simulink model "vnsimulink"  (R2020a)
settings: Solver=ode4  StartTime=0.0  StopTime=20  FixedStep=8e-6  RelTol=1e-3
undefined symbols (not defined in the file or in its folder): D1, Delta, sigbuilder_block
libraries: powerlib x98, powerlib_meascontrol x21, simulink x16
(part 3 of 3)

== system vnsimulink/PV15kW2/Subsystem/Subsystem/Power Loop2 ==
  vp : Inport
  vn : Inport  Port=2
  av : Inport  Port=3
  ip : Inport  Port=4
  outn : Inport  Port=5
  Trigger : TriggerPort  VariantControl=(inherit)
  Pcut-sim1 : MATLAB Function  TreatAsAtomicUnit=on
  Pmax-sim2 : MATLAB Function  TreatAsAtomicUnit=on
  Scope : Scope
  m : Outport
  m2 : Outport  Port=2
  m3 : Outport  Port=3
  m4 : Outport  Port=4
  wires:
  vp/1 -> Pmax-sim2/1(vp)
  vn/1 -> Pmax-sim2/2(vn)
  av/1 -> Pmax-sim2/3(av)
  ip/1 -> Pmax-sim2/4(ip)
  outn/1 -> Pmax-sim2/5(outn)
  Pmax-sim2/1(gn) -> m/1
  Pmax-sim2/2(phi) -> m2/1
  Pmax-sim2/3(kii) -> m3/1
  Pmax-sim2/4(ppv) -> m4/1
  Pmax-sim2/5(x) -> Scope/1

== system vnsimulink/PV15kW2/Subsystem/Subsystem2/integral  ==
  di : Inport
  kii : Inport  Port=2
  gmax : Inport  Port=3
  Trigger : TriggerPort  VariantControl=(inherit)
  Embedded MATLAB Function : MATLAB Function  TreatAsAtomicUnit=on
  w : Outport
  wires:
  Embedded MATLAB Function/1(w) -> w/1
  di/1 -> Embedded MATLAB Function/1(di)
  kii/1 -> Embedded MATLAB Function/2(kii)
  gmax/1 -> Embedded MATLAB Function/3(gmax)

== system vnsimulink/PV15kW2/Subsystem/Subsystem8/GIVF ==
  Vgq : Inport
  Trigger : TriggerPort  VariantControl=(inherit)
  Embedded MATLAB Function : MATLAB Function  TreatAsAtomicUnit=on
  Out1 : Outport
  y2 : Outport  Port=2
  wires:
  Embedded MATLAB Function/1(y1) -> Out1/1
  Vgq/1 -> Embedded MATLAB Function/1(u)
  Embedded MATLAB Function/2(y2) -> y2/1

== system vnsimulink/PV15kW2/Subsystem/Subsystem9/GIVF ==
  Vgq : Inport
  Trigger : TriggerPort  VariantControl=(inherit)
  Embedded MATLAB Function : MATLAB Function  TreatAsAtomicUnit=on
  Out1 : Outport
  y2 : Outport  Port=2
  wires:
  Embedded MATLAB Function/1(y1) -> Out1/1
  Vgq/1 -> Embedded MATLAB Function/1(u)
  Embedded MATLAB Function/2(y2) -> y2/1

== matlab function vnsimulink/PV15kW2/Subsystem/Subsystem/Power Loop2/Pcut-sim1 ==
  data: vp input; vn input; av input; gn output; phi output; ip input; outn input; kii output; ppv output
function [gn,phi,kii,ppv] = Algorithm(vp,vn,av,ip,outn)

ilim=41;
d=0.6;ppv=15060;
persistent flag D Dold ppvold ppv1
persistent ca ir i ki ctc
persistent m sum1 sum2 ipo an
persistent vns vps up un un0 un1 uns kn kn0 kns kn1 
persistent outns outn0 outn1 on m1 m2
persistent a1 b1 c1 a2 b2 c2 a3 b3 c3 kna knb knc A B C 
dataType = 'double';
%initial
if isempty(D)
flag=1;D=1;Dold=1;
ca=0;ir=0;i=0;ctc=0;
ipo=0;m=0;sum1=40;sum2=14;an=0;
vns=0;vps=0;ppvold=15000;ppv1=15000;
un=0;un0=0;un1=0;uns=0;kn=0;kn0=0;kns=0;kn1=0;
outns=0;outn0=0;outn1=0;on=0;m1=0;m2=0;ki=1;
a1=0;b1=0;c1=0;a2=0;b2=0;c2=0;a3=0;b3=0;c3=0;kna=0;knb=0;knc=0;A=0;B=0;C=0;
end
ctc=ctc+1;

if sum1>0
    sum1=sum1-1;
    vns=vns+vn;vps=vps+vp;
end
if sum1==0
sum1=40;
% vns=vns+vn;vps=vps+vp;
un=vns/40;up=vps/40;
vns=0;vps=0;

% no p limit
if flag==1
    un1=un;flag=0;kn=0;m=185;
else
    
if sum2==0
    sum2=14;
    un0=(uns+un)/11;
    outn0=(outns+outn)/11;
    kn0=(kns+kn)/11;

%PV power change?
  if (abs(ip-ipo)>0.1)
  ir=1;
  else
  ir=0;
  end
%select case
ca=0;ki=1;
if (ir==0)
  if (on==1)
      ca=1;end
  if (on==0)   
      ca=2;end 
  if (outn<kn)&&(un0<1.63)
      ca=3;end
%case1 
  if (ca==1)
   %power curtail
   vnx=2;
   zn=0.368;thv=37;vn0=7.11;
   if ctc>30600
   zn=0.373;thv=42.5;vn0=7.61;end
   if ctc>81000
   zn=0.4068;thv=43.4;vn0=8.27;end   
   %mp=th2-th1+atan(0.65)-pi;
   ipm=sqrt((ilim*zn+vnx)^2-(vn0*sin(thv/180*pi))^2)-vn0*cos(thv/180*pi);
   ppvn=1.5*ipm/zn*vp-1.5*vn*vn*kn;
   th1=pi-asin(vn0*sin(thv/180*pi)/(ilim*zn+vnx));
   xp=-ilim*zn/(sqrt(1+(vn0*sin(thv/180*pi)/(ilim*zn+vnx))^2));
   yp=-xp*vn0*sin(thv/180*pi)/(ilim*zn+vnx);
   th2=2*pi-atan(yp/(-xp-ipm));
   mp=th2-2/3*pi; 
   %exit curtail
    if abs(ppvold-ppvn)<75
    ppvn=ppvold;
    else
    m=mp*180/pi;
    ca=0;
    end
    ppv1=ppvn;
    ppvold=ppv1;
  end
  if (ca==1)    
   if Dold==1
    if un0>un1
      D=-1;
    else
      D=1;
    end
   else
    if un0>un1
      D=1;
    else
      D=-1;
    end 
   end
  end
%case2 
  if ca==2
    if (un0>1.003*un1)
    ca=2;ki=0;
    else
    ca=0;    
    end
  end
%case3
 if (ca==3)
  if Dold==1
   if un0*outn0>un1*outn1
      D=-1;
   else
      D=1;
   end
  else
   if un0*outn0>un1*outn1
      D=1;
   else
      D=-1;
   end 
  end
 end
%update D
 if (ca==1)||(ca==2)||(ca==3)
  Dold=D;
   if D==-1   
      m=m-d;
   else
      m=m+d;
   end
  end  
end
%%exit case
 un1=un0;outn1=outn0;kn1=kn0;ipo=ip;m2=m1;m1=m;
%%sum!=0
else
    if (sum2<=10)
        i=1;
    else
        i=2;
        if (sum2>10)
        i=0;
        end
    end
    if i==1
    uns=uns+un;outns=outns+outn;kns=kns+kn;sum2=sum2-1;i=3;
     if outn>kn
        on=1;end
    end
    if i==0
    uns=0;outns=0;kns=0;sum2=sum2-1;i=3;on=0;
     if outn>kn
        on=1;end
    end
    if i==2
    sum2=sum2-1;i=3;
     if outn>kn
        on=1;
     end
    end
end

%%current limit
     an=m/180*pi;
    a1=vn^2;
    b1=2*ip*un*cos(an);
    c1=ip^2-ilim^2;
kna=(-b1+sqrt(b1^2-4*a1*c1))/(2*a1);
    a3=vn^2;
    b3=2*ip*un*cos(an-pi*2/3);
    c3=ip^2-ilim^2;
knc=(-b3+sqrt(b3^2-4*a3*c3))/(2*a3);
    a2=vn^2;
    b2=2*ip*un*cos(an+pi*2/3);
    c2=ip^2-ilim^2;
knb=(-b2+sqrt(b2^2-4*a2*c2))/(2*a2);
kn=min(min(kna,knb),knc);
%power fluctuation
A=un^2*up^2;
B=2*un*up*ip*cos(av-an);
C=un^2*ip^2-(8000/1.5)^2;
knm=(-B+sqrt(B^2-4*A*C))/(2*A);
kn=min(kn,knm);
end
end
phi=m;gn=kn;kii=ki;ppv=ppv1;

== matlab function vnsimulink/PV15kW2/Subsystem/Subsystem2/integral /Embedded MATLAB Function ==
  data: di input; w output; kii input; gmax input
function w  = Algorithm(di,kii,gmax)

%控制器参数
T=20e-5;%控制周期
% ki1=3;
% ki2=3;
ki1=2.5;
ki2=12;
persistent sum ct;
dataType = 'double';

%首次赋值
if isempty(sum)
    sum=0;ct=0;
end

 if di>=0.2
 sum=kii*ki1*T*di+sum;
 else
 sum=kii*ki2*T*di+sum; 
 end
 
 if sum>1.1*gmax
     ct=ct+1;
     if ct==600
     ct=0;
     sum=1.07*gmax;
     end
 end   
   w=sum;

== matlab function vnsimulink/PV15kW2/Subsystem/Subsystem8/GIVF/Embedded MATLAB Function ==
  data: u input; y1 output; y2 output
function [y1,y2] = Algorithm(u)

%控制器参数
T=2e-4;k=314.1593;
persistent u0 u1 u2 u3 u4 u5;
dataType = 'double';

%首次赋值
if isempty(u0)
u0=0;u1=0;u2=0;u3=0;u4=0;u5=0;
end

u0=u;
u1=u0-u2-u3-u4;
u2=k*T*u1+u2;
u3=k*T*u2+u3;
u4=k*T*(0.5*u2-u5)+u4;
u5=k*T*u4+u5;
y1=0.5*u4;
y2=0.5*u5;
end

== matlab function vnsimulink/PV15kW2/Subsystem/Subsystem9/GIVF/Embedded MATLAB Function ==
  data: u input; y1 output; y2 output
function [y1,y2] = Algorithm(u)

%控制器参数
T=2e-4;k=314.1593;
persistent u0 u1 u2 u3 u4 u5;
dataType = 'double';

%首次赋值
if isempty(u0)
u0=0;u1=0;u2=0;u3=0;u4=0;u5=0;
end

u0=u;
u1=u0-u2-u3-u4;
u2=k*T*u1+u2;
u3=k*T*u2+u3;
u4=k*T*(0.5*u2-u5)+u4;
u5=k*T*u4+u5;
y1=0.5*u4;
y2=0.5*u5;
end

== matlab function vnsimulink/PV15kW2/Subsystem4/Power Loop1/Embedded MATLAB Function ==
  data: Vpv input; Ppv input; v output; l output; Pref input
function [v,l]= Algorithm(Vpv,Ppv,Pref)

%MPPT控制参数
v0 = 400;
vmax  = 600;
vmin = 200;
Deltav =0.1;


persistent Vpv_old Ppv_old v_old;
persistent flag nsum;


dataType = 'double';

%首次赋值
if isempty(Vpv_old)
    Vpv_old=0;
    Ppv_old=0;
    v_old=v0;
    flag=0;
    nsum=0;
end
% if nsum<(1.0/(20e-5))
%      flag=0;
% else
%      flag=1;
% end
% nsum=nsum+1;
% 
% if Vpv>800
%     flag=1;
% end
flag=1;
l=0;
if flag==1
%MPPT控制
dVpv=Vpv-Vpv_old;
dPpv=Ppv-Ppv_old;
if Ppv-Pref >= 0
    if dPpv >= 0
        if dVpv >= 0
            v = v_old + Deltav;%右侧
            l=11;
        else 
            v = v_old + Deltav;
            l=12;
        end
    else
        if dVpv >= 0
            v = v_old + Deltav;
            l=13;
        else
            v = v_old + Deltav;%右侧
            l=14;
        end
    end
else
    if dPpv >= 0
        if dVpv >=0
            v = v_old + Deltav;
             l=21;
        else
            v = v_old - Deltav;
             l=22;
        end
    else
        if dVpv >= 0
            v = v_old - Deltav;
             l=23;
        else
            v = v_old + Deltav;
             l=24;
        end
    end
end
% if Ppv-Pref >= 0
%      v = v_old - Deltav;
% else
%      v = v_old + Deltav;
% end
v_old=v;
Vpv_old=Vpv;
Ppv_old=Ppv;
else
 v=v0;   
end

== matlab function vnsimulink/PV15kW1/Subsystem/PLL/Embedded MATLAB Function ==
  data: Vgq input; w output
function w  = Algorithm(Vgq)

%控制器参数
T=20e-5;%控制周期

Kpllp=0.45;
Kplli=8;

persistent PLLsum;
persistent nsum2;

dataType = 'double';

%首次赋值
if isempty(PLLsum)
    PLLsum=0;
    nsum2=0;
end


w=Kpllp*Vgq+Kplli*(T*Vgq+PLLsum);
PLLsum=T*Vgq+PLLsum;
end

== matlab function vnsimulink/PV15kW2/Subsystem/PLL/Embedded MATLAB Function ==
  data: Vgq input; w output
function w  = Algorithm(Vgq)

%控制器参数
T=20e-5;%控制周期

Kpllp=0.45;
Kplli=8;

persistent PLLsum;
persistent nsum2;

dataType = 'double';

%首次赋值
if isempty(PLLsum)
    PLLsum=0;
    nsum2=0;
end


w=Kpllp*Vgq+Kplli*(T*Vgq+PLLsum);
PLLsum=T*Vgq+PLLsum;
end

== matlab function vnsimulink/PV15kW1/Subsystem/Subsystem/Power Loop2/Pcut-sim2 ==
  data: vp input; vn input; av input; gn output; phi output; ip input; outn input; kii output; ppv output
function [gn,phi,kii,ppv] = Algorithm(vp,vn,av,ip,outn)

ilim=41;
d=0.6;ppv=15060;
persistent flag D Dold ppvold ppv1
persistent ca ir i ki ctc
persistent m sum1 sum2 ipo an
persistent vns vps up un un0 un1 uns kn kn0 kns kn1 
persistent outns outn0 outn1 on m1 m2
persistent a1 b1 c1 a2 b2 c2 a3 b3 c3 kna knb knc A B C 
dataType = 'double';
%initial
if isempty(D)
flag=1;D=1;Dold=1;
ca=0;ir=0;i=0;ctc=0;
ipo=0;m=0;sum1=40;sum2=14;an=0;
vns=0;vps=0;ppvold=15000;ppv1=15000;
un=0;un0=0;un1=0;uns=0;kn=0;kn0=0;kns=0;kn1=0;
outns=0;outn0=0;outn1=0;on=0;m1=0;m2=0;ki=1;
a1=0;b1=0;c1=0;a2=0;b2=0;c2=0;a3=0;b3=0;c3=0;kna=0;knb=0;knc=0;A=0;B=0;C=0;
end
ctc=ctc+1;

if sum1>0
    sum1=sum1-1;
    vns=vns+vn;vps=vps+vp;
end
if sum1==0
sum1=40;
% vns=vns+vn;vps=vps+vp;
un=vns/40;up=vps/40;
vns=0;vps=0;

% no p limit
if flag==1
    un1=un;flag=0;kn=0;m=185;
else
    
if sum2==0
    sum2=14;
    un0=(uns+un)/11;
    outn0=(outns+outn)/11;
    kn0=(kns+kn)/11;

%PV power change?
  if (abs(ip-ipo)>0.1)
  ir=1;
  else
  ir=0;
  end
%select case
ca=0;ki=1;
if (ir==0)
  if (on==1)
      ca=1;end
  if (on==0)   
      ca=2;end 
  if (outn<kn)&&(un0<1.63)
      ca=3;end
%case1 
  if (ca==1)
   %power curtail
   vnx=2;
   zn=0.368;thv=37;vn0=7.11;
   if ctc>30600
   zn=0.373;thv=42.5;vn0=7.61;end
   if ctc>81000
   zn=0.4068;thv=43.4;vn0=8.27;end   
   %mp=th2-th1+atan(0.65)-pi;
   ipm=sqrt((ilim*zn+vnx)^2-(vn0*sin(thv/180*pi))^2)-vn0*cos(thv/180*pi);
   ppvn=1.5*ipm/zn*vp-1.5*vn*vn*kn;
   th1=pi-asin(vn0*sin(thv/180*pi)/(ilim*zn+vnx));
   xp=-ilim*zn/(sqrt(1+(vn0*sin(thv/180*pi)/(ilim*zn+vnx))^2));
   yp=-xp*vn0*sin(thv/180*pi)/(ilim*zn+vnx);
   th2=2*pi-atan(yp/(-xp-ipm));
   mp=th2-2/3*pi; 
   %exit curtail
    if abs(ppvold-ppvn)<75
    ppvn=ppvold;
    else
    m=mp*180/pi;
    ca=0;
    end
    ppv1=ppvn;
    ppvold=ppv1;
  end
  if (ca==1)    
   if Dold==1
    if un0>un1
      D=-1;
    else
      D=1;
    end
   else
    if un0>un1
      D=1;
    else
      D=-1;
    end 
   end
  end
%case2 
  if ca==2
    if (un0>1.003*un1)
    ca=2;ki=0;
    else
    ca=0;    
    end
  end
%case3
 if (ca==3)
  if Dold==1
   if un0*outn0>un1*outn1
      D=-1;
   else
      D=1;
   end
  else
   if un0*outn0>un1*outn1
      D=1;
   else
      D=-1;
   end 
  end
 end
%update D
 if (ca==1)||(ca==2)||(ca==3)
  Dold=D;
   if D==-1   
      m=m-d;
   else
      m=m+d;
   end
  end  
end
%%exit case
 un1=un0;outn1=outn0;kn1=kn0;ipo=ip;m2=m1;m1=m;
%%sum!=0
else
    if (sum2<=10)
        i=1;
    else
        i=2;
        if (sum2>10)
        i=0;
        end
    end
    if i==1
    uns=uns+un;outns=outns+outn;kns=kns+kn;sum2=sum2-1;i=3;
     if outn>kn
        on=1;end
    end
    if i==0
    uns=0;outns=0;kns=0;sum2=sum2-1;i=3;on=0;
     if outn>kn
        on=1;end
    end
    if i==2
    sum2=sum2-1;i=3;
     if outn>kn
        on=1;
     end
    end
end

%%current limit
     an=m/180*pi;
    a1=vn^2;
    b1=2*ip*un*cos(an);
    c1=ip^2-ilim^2;
kna=(-b1+sqrt(b1^2-4*a1*c1))/(2*a1);
    a3=vn^2;
    b3=2*ip*un*cos(an-pi*2/3);
    c3=ip^2-ilim^2;
knc=(-b3+sqrt(b3^2-4*a3*c3))/(2*a3);
    a2=vn^2;
    b2=2*ip*un*cos(an+pi*2/3);
    c2=ip^2-ilim^2;
knb=(-b2+sqrt(b2^2-4*a2*c2))/(2*a2);
kn=min(min(kna,knb),knc);
%power fluctuation
A=un^2*up^2;
B=2*un*up*ip*cos(av-an);
C=un^2*ip^2-(8000/1.5)^2;
knm=(-B+sqrt(B^2-4*A*C))/(2*A);
kn=min(kn,knm);
end
end
phi=m;gn=kn;kii=ki;ppv=ppv1;

== matlab function vnsimulink/PV15kW1/Subsystem/Subsystem/Power Loop2/Pmax-sim1 ==
  data: vp input; vn input; av input; gn output; phi output; ip input; outn input; kii output; ppv output
function [gn,phi,kii,ppv] = Algorithm(vp,vn,av,ip,outn)

ilim=39;
d=0.6;ppv=15060;
persistent flag D Dold 
persistent ca ir i ki
persistent m sum1 sum2 ipo an
persistent vns vps up un un0 un1 uns kn kn0 kns kn1 
persistent outns outn0 outn1 on m1 m2
persistent a1 b1 c1 a2 b2 c2 a3 b3 c3 kna knb knc A B C 
dataType = 'double';
%initial
if isempty(D)
flag=1;D=1;Dold=1;
ca=0;ir=0;i=0;
ipo=0;m=0;sum1=39;sum2=14;an=0;
vns=0;vps=0;
un=0;un0=0;un1=0;uns=0;kn=0;kn0=0;kns=0;kn1=0;
outns=0;outn0=0;outn1=0;on=0;m1=0;m2=0;ki=1;
a1=0;b1=0;c1=0;a2=0;b2=0;c2=0;a3=0;b3=0;c3=0;kna=0;knb=0;knc=0;A=0;B=0;C=0;
end

if sum1>0
    sum1=sum1-1;
    vns=vns+vn;vps=vps+vp;
end
if sum1==0
sum1=39;
vns=vns+vn;vps=vps+vp;
un=vns/40;up=vps/40;
vns=0;vps=0;

% no p limit
if flag==1
    un1=un;flag=0;kn=0;m=-65;
else
    
if sum2==0
    sum2=14;
    un0=(uns+un)/11;
    outn0=(outns+outn)/11;
    kn0=(kns+kn)/11;

%PV power change?
  if (abs(ip-ipo)>0.1)
  ir=1;
  else
  ir=0;
  end
%select case
ca=0;ki=1;
if (ir==0)
  if (on==1)
%     if (on==1)&&(m2~=m1)
      ca=1;end
%   if (on==0)||((on==1)&&(m2==m1))
  if (on==0)   
      ca=2;end 
  if (outn<kn)&&(un0<1.63)
      ca=3;end
%case1 
  if (ca==1)    
   if Dold==1
    if un0>un1
      D=-1;
    else
      D=1;
    end
   else
    if un0>un1
      D=1;
    else
      D=-1;
    end 
   end
  end
%case2 
  if ca==2
    if (un0>1.003*un1)
    ca=2;ki=0;
    else
    ca=0;    
    end
  end
%case3
 if (ca==3)
  if Dold==1
   if un0*outn0>un1*outn1
      D=-1;
   else
      D=1;
   end
  else
   if un0*outn0>un1*outn1
      D=1;
   else
      D=-1;
   end 
  end
 end
%update D
 if (ca==1)||(ca==2)||(ca==3)
  Dold=D;
   if D==-1   
      m=m-d;
   else
      m=m+d;
   end
  end  
end
%%exit case
 un1=un0;outn1=outn0;kn1=kn0;ipo=ip;m2=m1;m1=m;
%%sum!=0
else
    if (sum2<=10)
        i=1;
    else
        i=2;
        if (sum2>10)
        i=0;
        end
    end
    if i==1
    uns=uns+un;outns=outns+outn;kns=kns+kn;sum2=sum2-1;i=3;
     if outn>kn
        on=1;end
    end
    if i==0
    uns=0;outns=0;kns=0;sum2=sum2-1;i=3;on=0;
     if outn>kn
        on=1;end
    end
    if i==2
    sum2=sum2-1;i=3;
     if outn>kn
        on=1;
     end
    end
end
%这一行是相对相角控制
% m=av*180/pi+180;
% m=-60;
%%current limit
     an=m/180*pi;
    a1=vn^2;
    b1=2*ip*un*cos(an);
    c1=ip^2-ilim^2;
kna=(-b1+sqrt(b1^2-4*a1*c1))/(2*a1);
    a3=vn^2;
    b3=2*ip*un*cos(an-pi*2/3);
    c3=ip^2-ilim^2;
knc=(-b3+sqrt(b3^2-4*a3*c3))/(2*a3);
    a2=vn^2;
    b2=2*ip*un*cos(an+pi*2/3);
    c2=ip^2-ilim^2;
knb=(-b2+sqrt(b2^2-4*a2*c2))/(2*a2);
kn=min(min(kna,knb),knc);
%power fluctuation
A=un^2*up^2;
B=2*un*up*ip*cos(av-an);
C=un^2*ip^2-(8000/1.5)^2;
knm=(-B+sqrt(B^2-4*A*C))/(2*A);
kn=min(kn,knm);
end
end
phi=m;gn=kn;kii=ki;

== matlab function vnsimulink/PV15kW1/Subsystem/Subsystem2/integral /Embedded MATLAB Function ==
  data: di input; w output; kii input; gmax input
function w  = Algorithm(di,kii,gmax)

%控制器参数
T=20e-5;%控制周期
% ki1=3;
% ki2=3;
ki1=2;
ki2=12;
persistent sum ct;
dataType = 'double';

%首次赋值
if isempty(sum)
    sum=0;ct=0;
end

 if di>=0.2
 sum=kii*ki1*T*di+sum;
 else
 sum=kii*ki2*T*di+sum; 
 end
 
 if sum>1.1*gmax
     ct=ct+1;
     if ct==600
     ct=0;
     sum=1.07*gmax;
     end
 end   
   w=sum;

== matlab function vnsimulink/PV15kW1/Subsystem4/Power Loop1/Embedded MATLAB Function ==
  data: Vpv input; Ppv input; v output; l output; Pref input
function [v,l]= Algorithm(Vpv,Ppv,Pref)

%MPPT控制参数
v0 = 400;
vmax  = 600;
vmin = 200;
Deltav =0.1;


persistent Vpv_old Ppv_old v_old;
persistent flag nsum;


dataType = 'double';

%首次赋值
if isempty(Vpv_old)
    Vpv_old=0;
    Ppv_old=0;
    v_old=v0;
    flag=0;
    nsum=0;
end
% if nsum<(1.0/(20e-5))
%      flag=0;
% else
%      flag=1;
% end
% nsum=nsum+1;
% 
% if Vpv>800
%     flag=1;
% end
flag=1;
l=0;
if flag==1
%MPPT控制
dVpv=Vpv-Vpv_old;
dPpv=Ppv-Ppv_old;
if Ppv-Pref >= 0
    if dPpv >= 0
        if dVpv >= 0
            v = v_old + Deltav;%右侧
            l=11;
        else 
            v = v_old + Deltav;
            l=12;
        end
    else
        if dVpv >= 0
            v = v_old + Deltav;
            l=13;
        else
            v = v_old + Deltav;%右侧
            l=14;
        end
    end
else
    if dPpv >= 0
        if dVpv >=0
            v = v_old + Deltav;
             l=21;
        else
            v = v_old - Deltav;
             l=22;
        end
    else
        if dVpv >= 0
            v = v_old - Deltav;
             l=23;
        else
            v = v_old + Deltav;
             l=24;
        end
    end
end
% if Ppv-Pref >= 0
%      v = v_old - Deltav;
% else
%      v = v_old + Deltav;
% end
v_old=v;
Vpv_old=Vpv;
Ppv_old=Ppv;
else
 v=v0;   
end

== matlab function vnsimulink/PV15kW2/Subsystem/Subsystem/Power Loop2/Pmax-sim2 ==
  data: vp input; vn input; av input; gn output; phi output; ip input; outn input; kii output; ppv output; x output
function [gn,phi,kii,ppv,x] = Algorithm(vp,vn,av,ip,outn)

ilim=41;
d=0.6;ppv=15060;
persistent flag D Dold 
persistent ca ir i ki
persistent m sum1 sum2 ipo an
persistent vns vps up un un0 un1 uns kn kn0 kns kn1 
persistent outns outn0 outn1 on m1 m2
persistent a1 b1 c1 a2 b2 c2 a3 b3 c3 kna knb knc A B C 
dataType = 'double';
%initial
if isempty(D)
flag=1;D=1;Dold=1;
ca=0;ir=0;i=0;
ipo=0;m=0;sum1=39;sum2=14;an=0;
vns=0;vps=0;
un=0;un0=0;un1=0;uns=0;kn=0;kn0=0;kns=0;kn1=0;
outns=0;outn0=0;outn1=0;on=0;m1=0;m2=0;ki=1;
a1=0;b1=0;c1=0;a2=0;b2=0;c2=0;a3=0;b3=0;c3=0;kna=0;knb=0;knc=0;A=0;B=0;C=0;
end

if sum1>0
    sum1=sum1-1;
    vns=vns+vn;vps=vps+vp;
end
if sum1==0
sum1=39;%原39应为40
vns=vns+vn;vps=vps+vp;
un=vns/40;up=vps/40;
vns=0;vps=0;

% no p limit
if flag==1
    un1=un;flag=0;kn=0;m=180;%270-0.8，290-0.8，240-0.6
else
    
if sum2==0
    sum2=13;
    un0=(uns+un)/10;
    outn0=(outns+outn)/10;
    kn0=(kns+kn)/10;

%PV power change?
  if (abs(ip-ipo)>0.1)
  ir=1;
  else
  ir=0;
  end
%select case
ca=0;ki=1;
if (ir==0)
  if (on==1)
%     if (on==1)&&(m2~=m1)
      ca=1;end
%   if (on==0)||((on==1)&&(m2==m1))
  if (on==0)   
      ca=2;end 
  if (outn<kn)&&(un0<1.63)
      ca=3;end
%case1 
  if (ca==1)    
   if Dold==1
    if un0>un1
      D=-1;
    else
      D=1;
    end
   else
    if un0>un1
      D=1;
    else
      D=-1;
    end 
   end
  end
%case2 
  if ca==2
    if (un0>1.003*un1)
    ca=2;ki=0;
    else
    ca=0;    
    end
  end
%case3
 if (ca==3)
  if Dold==1
   if un0*outn0>un1*outn1
      D=-1;
   else
      D=1;
   end
  else
   if un0*outn0>un1*outn1
      D=1;
   else
      D=-1;
   end 
  end
 end
%update D
 if (ca==1)||(ca==2)||(ca==3)
  Dold=D;
   if D==-1   
      m=m-d;
   else
      m=m+d;%4-1都用减号
   end
  end  
end
%%exit case
 un1=un0;outn1=outn0;kn1=kn0;ipo=ip;m2=m1;m1=m;
%%sum!=0
else
    if (sum2<=9)
        i=1;
    else
        i=2;
        if (sum2>9)
        i=0;
        end
    end
    if i==1
    uns=uns+un;outns=outns+outn;kns=kns+kn;sum2=sum2-1;i=3;
     if outn>kn
        on=1;end
    end
    if i==0
    uns=0;outns=0;kns=0;sum2=sum2-1;i=3;on=0;
     if outn>kn
        on=1;end
    end
    if i==2
    sum2=sum2-1;i=3;
     if outn>kn
        on=1;
     end
    end
end
%这一行是相对相角控制
% m=av*180/pi+180;
% m=180;
%%current limit
     an=m/180*pi;
    a1=vn^2;
    b1=2*ip*un*cos(an);
    c1=ip^2-ilim^2;
kna=(-b1+sqrt(b1^2-4*a1*c1))/(2*a1);
    a3=vn^2;
    b3=2*ip*un*cos(an-pi*2/3);
    c3=ip^2-ilim^2;
knc=(-b3+sqrt(b3^2-4*a3*c3))/(2*a3);
    a2=vn^2;
    b2=2*ip*un*cos(an+pi*2/3);
    c2=ip^2-ilim^2;
knb=(-b2+sqrt(b2^2-4*a2*c2))/(2*a2);
kn=min(min(kna,knb),knc);
%power fluctuation
A=un^2*up^2;
B=2*un*up*ip*cos(av-an);
C=un^2*ip^2-(8000/1.5)^2;
knm=(-B+sqrt(B^2-4*A*C))/(2*A);
kn=min(kn,knm);
end
end
phi=m;gn=kn;kii=ki;x=ca;
